simulink model "Simulink"  (R2017a)
settings: Solver=VariableStepAuto  StartTime=0.0  StopTime=60  RelTol=1e-3  EnableMultiTasking=on
values from neighbouring files (symbols this model uses):
  K_i = K_da(5)    [Matlab.m]
  L_d = (place(A_d',C',p_ed))'    [Matlab.m]
  N_d = 1/(C_d*inv(I-A_d+B_d*K)*B_d )    [Matlab.m]
  T_sample = 0.0001    [Matlab.m]
undefined symbols (not defined in the file or in its folder): A_d, B_d, C_d
libraries: simulink x2
settings Model: Creator=apfausto  LastModifiedBy=PURVANG
settings DataIOCC: LimitDataPoints=on
settings OptimizationCC: LifeSpan=inf
settings DebuggingCC: AllowSymbolicDim=off  SFUnexpectedBacktrackingDiag=warning  SFNoUnconditionalDefaultTransitionDiag=warning  SFExecutionAtInitializationDiag=none
settings ModelReferenceCC: PropagateSignalLabelsOutOfModel=off
settings GRTTargetCC: TargetLangStandard=C89/C90 (ANSI)
settings ConfigComp: CovMetricSettings=dw  CovHtmlReporting=on  CovSaveCumulativeToWorkspaceVar=on  CovSaveSingleToWorkspaceVar=on  CovExternalEMLEnable=off

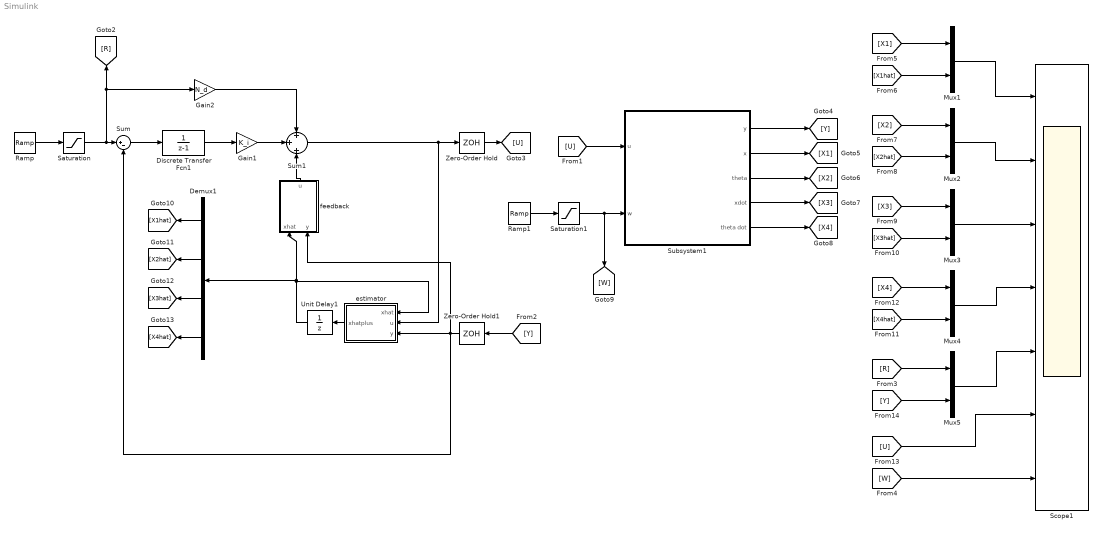
== system Simulink ==
  Demux1 : Demux
  Discrete Transfer Fcn1 : DiscreteTransferFcn  Denominator=[1 -1]  SampleTime=T_sample
  Gain1 : Gain  Gain=K_i
  Gain2 : Gain  Gain=N_d
  Mux{1..5} (5 alike) : Mux  Inputs=2
  Ramp : simulink/Sources/Ramp  slope=0.01  start=10  X0=0
  Ramp1 : simulink/Sources/Ramp  slope=0.01  start=40  X0=0
  Saturation : Saturate  UpperLimit=0.25
  Saturation1 : Saturate  UpperLimit=0.1
  Scope1 : Scope  NumInputPorts=7
  Subsystem1 : Subsystem
  Sum : Sum  Inputs=|+-
  Sum1 : Sum  Inputs=+|+|+
  Unit Delay1 : UnitDelay  InitialCondition=[0 0 0 0]  SampleTime=T_sample
  Zero-Order Hold : ZeroOrderHold  SampleTime=T_sample
  Zero-Order Hold1 : ZeroOrderHold  SampleTime=T_sample
  estimator : MATLAB Function  TreatAsAtomicUnit=on
  feedback : MATLAB Function  TreatAsAtomicUnit=on
  wires:
  Saturation/1 -> Gain2/1, [R], Sum/1
  Sum/1 -> Discrete Transfer Fcn1/1
  Discrete Transfer Fcn1/1 -> Gain1/1
  Gain1/1 -> Sum1/2
  Gain2/1 -> Sum1/1
  Sum1/1 -> estimator/2(u), Zero-Order Hold/1
  Zero-Order Hold/1 -> [U]
  Subsystem1/5(theta dot) -> [X4]
  [U] -> Subsystem1/1(u)
  Subsystem1/1(y) -> [Y]
  Subsystem1/2(x) -> [X1]
  Subsystem1/3(theta) -> [X2]
  Subsystem1/4(xdot) -> [X3]
  Saturation1/1 -> Subsystem1/2("w "), [W]
  estimator/1(xhatplus) -> Unit Delay1/1
  Zero-Order Hold1/1 -> estimator/3(y), Sum/2, feedback/2(y)
  [Y] -> Zero-Order Hold1/1
  Unit Delay1/1 -> feedback/1(xhat), Demux1/1, estimator/1(xhat)
  Demux1/1 -> [X1hat]
  Demux1/2 -> [X2hat]
  Demux1/3 -> [X3hat]
  Demux1/4 -> [X4hat]
  feedback/1(u) -> Sum1/3
  Mux1/1 -> Scope1/1
  Mux2/1 -> Scope1/2
  Mux4/1 -> Scope1/4
  Mux3/1 -> Scope1/3
  [R] -> Mux5/1
  [W] -> Scope1/7
  [X1] -> Mux1/1
  [X1hat] -> Mux1/2
  [X2] -> Mux2/1
  [X2hat] -> Mux2/2
  [X3] -> Mux3/1
  [X3hat] -> Mux3/2
  [X4] -> Mux4/1
  [X4hat] -> Mux4/2
  [U] -> Scope1/6
  [Y] -> Mux5/2
  Mux5/1 -> Scope1/5
  Ramp/1 -> Saturation/1
  Ramp1/1 -> Saturation1/1

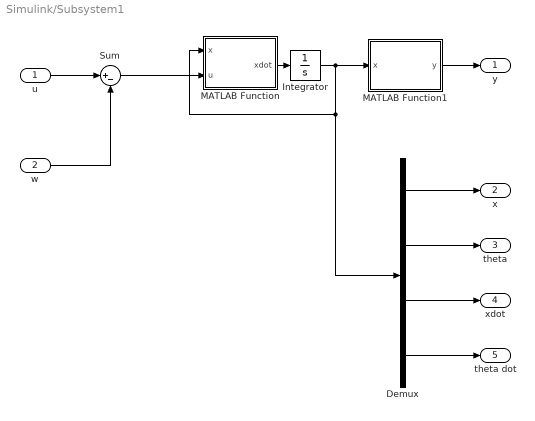
== system Simulink/Subsystem1 ==
  u : Inport
  "w " : Inport  Port=2
  Demux : Demux
  Integrator : Integrator  InitialCondition="[0.0  0.01  0.0  0.0]"
  MATLAB Function : MATLAB Function  TreatAsAtomicUnit=on
  MATLAB Function1 : MATLAB Function  TreatAsAtomicUnit=on
  Sum : Sum  Inputs=|+-
  y : Outport
  x : Outport  Port=2
  theta : Outport  Port=3
  xdot : Outport  Port=4
  theta dot : Outport  Port=5
  wires:
  u/1 -> Sum/1
  "w "/1 -> Sum/2
  MATLAB Function1/1(y) -> y/1
  Integrator/1 -> Demux/1, MATLAB Function/1(x), MATLAB Function1/1(x)
  Demux/4 -> theta dot/1
  Demux/3 -> xdot/1
  Demux/2 -> theta/1
  Demux/1 -> x/1
  MATLAB Function/1(xdot) -> Integrator/1
  Sum/1 -> MATLAB Function/2(u)

== matlab function Simulink/feedback ==
  data: u output size=1; K parameter size=[1,4]; xhat input size=4; y input size=1
function u=feedback(K,xhat,y)

u=-(K(1)*y + K(2)*xhat(2) + K(3)*xhat(3) + K(4)*xhat(4));

end

== matlab function Simulink/estimator ==
  data: A_d parameter size=[4,4]; B_d parameter size=[4,1]; C_d parameter size=[1,4]; xhat input size=4; u input size=1; L_d parameter size=[4,1]; y input size=1; xhatplus output size=4
function xhatplus=estimator(A_d, B_d, C_d, xhat, u, L_d,y)

    xhatplus= A_d*xhat + B_d*u + L_d*(y - C_d*xhat);
end

== matlab function Simulink/Subsystem1/MATLAB Function ==
  data: x input size=4; u input size=1; xdot output size=4
function xdot=invp_dyn(x,u)

% Define the non linear dynamic model for inverted pendulum
% in xdot = f(x,y;t) form

% Parameters of the model

m1 = 1.0 ;
m2 = 1.0 ;
l = 10.0 ;
g = 10.0 ;
% State Vector: [x(1) x(2) x(3) x(4) ] = [x theta xdot thetadot ]

J = [ (m1+m2) 0.5*m2*l*cos(x(2))
0.5*m2*l*cos(x(2)) (1.0/3.0)*m2*(l^2) ] ;

detJ = J(1,1)*J(2,2) - J(1,2)*J(2,1) ;

invJ = [ J(2,2)/detJ -J(2,1)/detJ
        -J(1,2)/detJ J(1,1)/detJ ]' ;
    
temp = invJ * [ 0.5*m2*l*(x(4)^2)*sin(x(2))+ u
                0.5*m2*g*l*sin(x(2)) ];
            
xdot = [ x(3)
         x(4)
         temp(1)
         temp(2) ] ;
return ;

== matlab function Simulink/Subsystem1/MATLAB Function1 ==
  data: C parameter size=[1,4]; y output size=1; x input size=4
function y = output(C,x)

    y=C*x;
    
end
